simulink model "task1_signal_u_func"  (R2021b)
settings: Solver=FixedStepAuto  StartTime=0.0  StopTime=3  FixedStep=0.0001  RelTol=1e-3
settings Model: Creator=den  LastModifiedBy=den

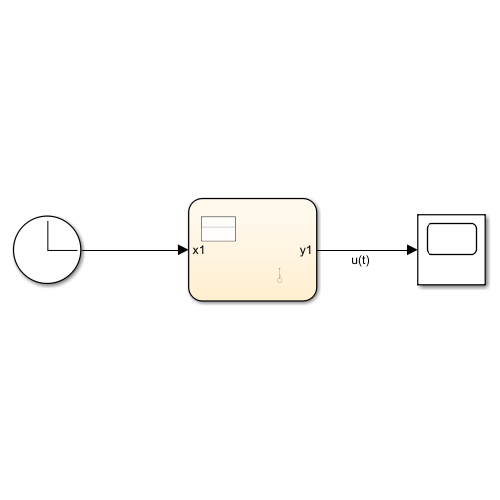
[thumbnail: Simulink's stored preview of the top-level diagram]
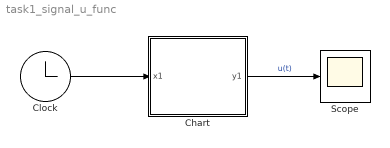
== system task1_signal_u_func ==
  Chart : Stateflow chart  TreatAsAtomicUnit=on
  Clock : Clock
  Scope : Scope
  wires:
  Clock/1 -> Chart/1(x1)
  Chart/1(y1) -> Scope/1  "u(t)"

== matlab function task1_signal_u_func/Chart ==
  data: x function_input; y function_output; x1 input; y1 output
function y = u(x)
    y = -0.002446 .* exp(3 .* x) + 2.7183 .^ x .* (0.734 .* cos(6 - 2 .* x) + 0.1772 .* sin(6 - 2 .* x));
end
